simulink model "gm_NewSignalGenerator"  (R2026a)
settings: Solver=VariableStepAuto  StopTime=20e-4
libraries: dsphdlxfrm2 x1, simulink x1
settings Model: Creator=adams
settings OptimizationCC: ConditionallyExecuteInputs=off
settings DebuggingCC: InheritedTsInSrcMsg=none

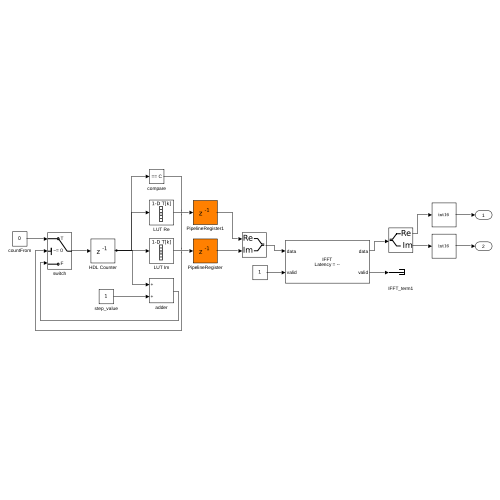
[thumbnail: Simulink's stored preview of the top-level diagram]
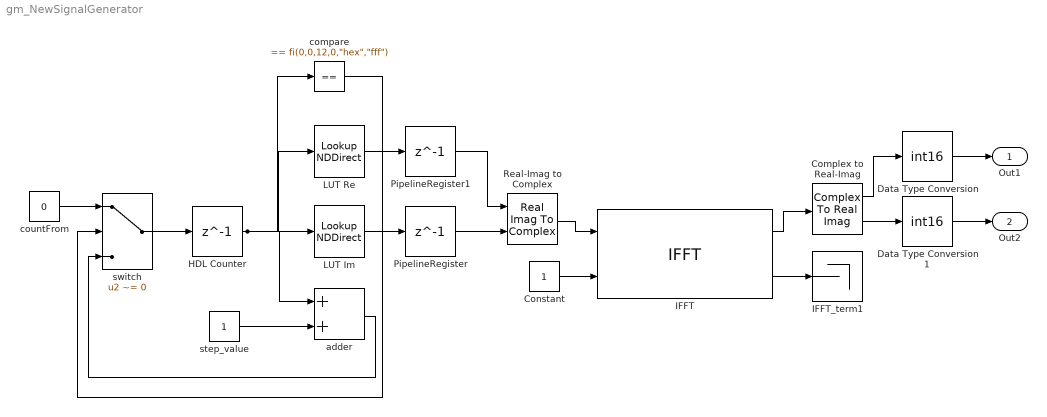
== system gm_NewSignalGenerator ==
  Complex to Real-Imag : ComplexToRealImag  SampleTime=6.51041666666667e-09
  Constant : Constant  OutDataTypeStr=boolean  SampleTime=6.51041666666667e-09
  Data Type Conversion : DataTypeConversion  OutDataTypeStr=int16  SampleTime=6.51041666666667e-09  SaturateOnIntegerOverflow=off  RndMeth=Floor
  Data Type Conversion1 : DataTypeConversion  OutDataTypeStr=int16  SampleTime=6.51041666666667e-09  SaturateOnIntegerOverflow=off  RndMeth=Floor
  HDL Counter : Delay  DelayLength=1  InitialCondition=0  SampleTime=6.51041666666667e-09
  IFFT : dsphdlxfrm2/IFFT  Architecture=Streaming Radix 2^2  FFTLengthSource=Property  FFTLength=4096  FFTLengthMax=1024  ComplexMultiplication=Use 4 multipliers and 2 adders  BitReversedOutput=off  BitReversedInput=off  Normalize=off  SimulateUsing=Code generation  RoundingMethod=Floor  ResetInputPort=off  StartOutputPort=off  EndOutputPort=off
  IFFT_term1 : Terminator
  LUT Im : LookupNDDirect  NumberOfTableDimensions=1  Table="reshape(double([0;0;0;0;0;0;0;0;-9;0;0;0;0;0;0;0;35;0;0;0;0;0;0;0;-78;0;0;0;0;0;0;0;138;0;0;0;0;0;0;0;-215;0;0;0;0;0;0;0;307;0;0;0;0;0;0;0;-413;0;0;0;0;0;0;0;530;0;0;0;0;0;0;0;-654;0;0;0;0;0;0;0;778;0;0;0;0;0;0;0;-895;0;0;0;0;0;0;0;995;0;0;0;0;0;0;0;-1068;0;0;0;0;0;0;0;1099;0;0;0;0;0;0;0;-1079;0;0;0;0;0;0;0;995;0;0;0;0;0;0;0;-842;0;0;0;0;0;0;0;618;0;0;0;0;0;0;0;-332;0;0;0;0;0;0;0;0;0;0;0;0;0;0;0;348;0;0;0;0;0;0;0;-674;0;0;0;0;0;0;0;933;0;0;0;0;0;0;0;-1081;0;0;0;0;0;0;0;1079;0;0;0;0;0;0;0;-910;0;0;0;0;0;0;0;582;0;0;0;0;0;0;0;-138;0;0;0;0;0;0;0;-348;0;0;0;0;0;0;0;778;0;0;0;0;0;0;0;-1049;0;0;0;0;0;0;0;1081;0;0;0;0;0;0;0;-842;0;0;0;0;0;0;0;373;0;0;0;0;0;0;0;215;0;0;0;0;0;0;0;-753;0;0;0;0;0;0;0;1068;0;0;0;0;0;0;0;-1035;0;0;0;0;0;0;0;640;0;0;0;0;0;0;0;0;0;0;0;0;0;0;0;-654;0;0;0;0;0;0;0;1056;0;0;0;0;0;0;0;-1020;0;0;0;0;0;0;0;530;0;0;0;0;0;0;0;215;0;0;0;0;0;0;0;-869;0;0;0;0;0;0;0;1097;0;0;0;0;0;0;0;-753;0;0;0;0;0;0;0;-9;0;0;0;0;0;0;0;778;0;0;0;0;0;0;0;-1100;0;0;0;0;0;0;0;753;0;0;0;0;0;0;0;78;0;0;0;0;0;0;0;-869;0;0;0;0;0;0;0;1079;0;0;0;0;0;0;0;-530;0;0;0;0;0;0;0;-413;0;0;0;0;0;0;0;1056;0;0;0;0;0;0;0;-885;0;0;0;0;0;0;0;0;0;0;0;0;0;0;0;895;0;0;0;0;0;0;0;-1035;0;0;0;0;0;0;0;265;0;0;0;0;0;0;0;753;0;0;0;0;0;0;0;-1079;0;0;0;0;0;0;0;373;0;0;0;0;0;0;0;708;0;0;0;0;0;0;0;-1081;0;0;0;0;0;0;0;332;0;0;0;0;0;0;0;778;0;0;0;0;0;0;0;-1043;0;0;0;0;0;0;0;138;0;0;0;0;0;0;0;933;0;0;0;0;0;0;0;-910;0;0;0;0;0;0;0;-215;0;0;0;0;0;0;0;1081;0;0;0;0;0;0;0;-582;0;0;0;0;0;0;0;-674;0;0;0;0;0;0;0;1043;0;0;0;0;0;0;0;0;0;0;0;0;0;0;0;-1049;0;0;0;0;0;0;0;618;0;0;0;0;0;0;0;708;0;0;0;0;0;0;0;-995;0;0;0;0;0;0;0;-215;0;0;0;0;0;0;0;1099;0;0;0;0;0;0;0;-265;0;0;0;0;0;0;0;-995;0;0;0;0;0;0;0;640;0;0;0;0;0;0;0;778;0;0;0;0;0;0;0;-885;0;0;0;0;0;0;0;-530;0;0;0;0;0;0;0;1020;0;0;0;0;0;0;0;307;0;0;0;0;0;0;0;-1079;0;0;0;0;0;0;0;-138;0;0;0;0;0;0;0;1097;0;0;0;0;0;0;0;35;0;0;0;0;0;0;0;-1100;0;0;0;0;0;0;0;0;0;0;0;0;0;0;0;1100;0;0;0;0;0;0;0;35;0;0;0;0;0;0;0;-1097;0;0;0;0;0;0;0;-138;0;0;0;0;0;0;0;1079;0;0;0;0;0;0;0;307;0;0;0;0;0;0;0;-1020;0;0;0;0;0;0;0;-530;0;0;0;0;0;0;0;885;0;0;0;0;0;0;0;778;0;0;0;0;0;0;0;-640;0;0;0;0;0;0;0;-995;0;0;0;0;0;0;0;265;0;0;0;0;0;0;0;1099;0;0;0;0;0;0;0;215;0;0;0;0;0;0;0;-995;0;0;0;0;0;0;0;-708;0;0;0;0;0;0;0;618;0;0;0;0;0;0;0;1049;0;0;0;0;0;0;0;0;0;0;0;0;0;0;0;-1043;0;0;0;0;0;0;0;-674;0;0;0;0;0;0;0;582;0;0;0;0;0;0;0;1081;0;0;0;0;0;0;0;215;0;0;0;0;0;0;0;-910;0;0;0;0;0;0;0;-933;0;0;0;0;0;0;0;138;0;0;0;0;0;0;0;1043;0;0;0;0;0;0;0;778;0;0;0;0;0;0;0;-332;0;0;0;0;0;0;0;-1081;0;0;0;0;0;0;0;-708;0;0;0;0;0;0;0;373;0;0;0;0;0;0;0;1079;0;0;0;0;0;0;0;753;0;0;0;0;0;0;0;-265;0;0;0;0;0;0;0;-1035;0;0;0;0;0;0;0;-895;0;0;0;0;0;0;0;0;0;0;0;0;0;0;0;885;0;0;0;0;0;0;0;1056;0;0;0;0;0;0;0;413;0;0;0;0;0;0;0;-530;0;0;0;0;0;0;0;-1079;0;0;0;0;0;0;0;-869;0;0;0;0;0;0;0;-78;0;0;0;0;0;0;0;753;0;0;0;0;0;0;0;1100;0;0;0;0;0;0;0;778;0;0;0;0;0;0;0;9;0;0;0;0;0;0;0;-753;0;0;0;0;0;0;0;-1097;0;0;0;0;0;0;0;-869;0;0;0;0;0;0;0;-215;0;0;0;0;0;0;0;530;0;0;0;0;0;0;0;1020;0;0;0;0;0;0;0;1056;0;0;0;0;0;0;0;654;0;0;0;0;0;0;0;0;0;0;0;0;0;0;0;-640;0;0;0;0;0;0;0;-1035;0;0;0;0;0;0;0;-1068;0;0;0;0;0;0;0;-753;0;0;0;0;0;0;0;-215;0;0;0;0;0;0;0;373;0;0;0;0;0;0;0;842;0;0;0;0;0;0;0;1081;0;0;0;0;0;0;0;1049;0;0;0;0;0;0;0;778;0;0;0;0;0;0;0;348;0;0;0;0;0;0;0;-138;0;0;0;0;0;0;0;-582;0;0;0;0;0;0;0;-910;0;0;0;0;0;0;0;-1079;0;0;0;0;0;0;0;-1081;0;0;0;0;0;0;0;-933;0;0;0;0;0;0;0;-674;0;0;0;0;0;0;0;-348;0;0;0;0;0;0;0;0;0;0;0;0;0;0;0;332;0;0;0;0;0;0;0;618;0;0;0;0;0;0;0;842;0;0;0;0;0;0;0;995;0;0;0;0;0;0;0;1079;0;0;0;0;0;0;0;1099;0;0;0;0;0;0;0;1068;0;0;0;0;0;0;0;995;0;0;0;0;0;0;0;895;0;0;0;0;0;0;0;778;0;0;0;0;0;0;0;654;0;0;0;0;0;0;0;530;0;0;0;0;0;0;0;413;0;0;0;0;0;0;0;307;0;0;0;0;0;0;0;215;0;0;0;0;0;0;0;138;0;0;0;0;0;0;0;78;0;0;0;0;0;0;0;35;0;0;0;0;0;0;0;9;0;0;0;0;0;0;0;0;0;0;0;0;0;0;0;0;0;0;0;0;0;0;0;0;0;0;0;0;0;0;0;0;0;0;0;0;0;0;0;0;0;0;0;0;0;0;0;0;0;0;0;0;0;0;0;0;0;0;0;0;0;0;0;0;0;0;0;0;0;0;0;0;0;0;0;0;0;0;0;0;0;0;0;0;0;0;0;0;0;0;0;0;0;0;0;0;0;0;0;0;0;0;0;0;0;0;0;0;0;0;0;0;0;0;0;0;0;0;0;0;0;0;0;0;0;0;0;0;0;0;0;0;0;0;0;0;0;0;0;0;0;0;0;0;0;0;0;0;0;0;0;0;0;0 ...(+5202 chars)]), [4096     1])"  SampleTime=6.51041666666667e-09  TableDataTypeStr=fixdt(1,32,20)
  LUT Re : LookupNDDirect  NumberOfTableDimensions=1  Table="reshape(double([1100;0;0;0;0;0;0;0;-1100;0;0;0;0;0;0;0;1099;0;0;0;0;0;0;0;-1097;0;0;0;0;0;0;0;1091;0;0;0;0;0;0;0;-1079;0;0;0;0;0;0;0;1056;0;0;0;0;0;0;0;-1020;0;0;0;0;0;0;0;964;0;0;0;0;0;0;0;-885;0;0;0;0;0;0;0;778;0;0;0;0;0;0;0;-640;0;0;0;0;0;0;0;468;0;0;0;0;0;0;0;-265;0;0;0;0;0;0;0;35;0;0;0;0;0;0;0;215;0;0;0;0;0;0;0;-468;0;0;0;0;0;0;0;708;0;0;0;0;0;0;0;-910;0;0;0;0;0;0;0;1049;0;0;0;0;0;0;0;-1100;0;0;0;0;0;0;0;1043;0;0;0;0;0;0;0;-869;0;0;0;0;0;0;0;582;0;0;0;0;0;0;0;-206;0;0;0;0;0;0;0;-215;0;0;0;0;0;0;0;618;0;0;0;0;0;0;0;-933;0;0;0;0;0;0;0;1091;0;0;0;0;0;0;0;-1043;0;0;0;0;0;0;0;778;0;0;0;0;0;0;0;-332;0;0;0;0;0;0;0;-206;0;0;0;0;0;0;0;708;0;0;0;0;0;0;0;-1035;0;0;0;0;0;0;0;1079;0;0;0;0;0;0;0;-802;0;0;0;0;0;0;0;265;0;0;0;0;0;0;0;373;0;0;0;0;0;0;0;-895;0;0;0;0;0;0;0;1100;0;0;0;0;0;0;0;-885;0;0;0;0;0;0;0;307;0;0;0;0;0;0;0;413;0;0;0;0;0;0;0;-964;0;0;0;0;0;0;0;1079;0;0;0;0;0;0;0;-674;0;0;0;0;0;0;0;-78;0;0;0;0;0;0;0;802;0;0;0;0;0;0;0;-1100;0;0;0;0;0;0;0;778;0;0;0;0;0;0;0;9;0;0;0;0;0;0;0;-802;0;0;0;0;0;0;0;1097;0;0;0;0;0;0;0;-674;0;0;0;0;0;0;0;-215;0;0;0;0;0;0;0;964;0;0;0;0;0;0;0;-1020;0;0;0;0;0;0;0;307;0;0;0;0;0;0;0;654;0;0;0;0;0;0;0;-1100;0;0;0;0;0;0;0;640;0;0;0;0;0;0;0;373;0;0;0;0;0;0;0;-1068;0;0;0;0;0;0;0;802;0;0;0;0;0;0;0;215;0;0;0;0;0;0;0;-1035;0;0;0;0;0;0;0;842;0;0;0;0;0;0;0;206;0;0;0;0;0;0;0;-1049;0;0;0;0;0;0;0;778;0;0;0;0;0;0;0;348;0;0;0;0;0;0;0;-1091;0;0;0;0;0;0;0;582;0;0;0;0;0;0;0;618;0;0;0;0;0;0;0;-1079;0;0;0;0;0;0;0;206;0;0;0;0;0;0;0;933;0;0;0;0;0;0;0;-869;0;0;0;0;0;0;0;-348;0;0;0;0;0;0;0;1100;0;0;0;0;0;0;0;-332;0;0;0;0;0;0;0;-910;0;0;0;0;0;0;0;842;0;0;0;0;0;0;0;468;0;0;0;0;0;0;0;-1079;0;0;0;0;0;0;0;35;0;0;0;0;0;0;0;1068;0;0;0;0;0;0;0;-468;0;0;0;0;0;0;0;-895;0;0;0;0;0;0;0;778;0;0;0;0;0;0;0;654;0;0;0;0;0;0;0;-964;0;0;0;0;0;0;0;-413;0;0;0;0;0;0;0;1056;0;0;0;0;0;0;0;215;0;0;0;0;0;0;0;-1091;0;0;0;0;0;0;0;-78;0;0;0;0;0;0;0;1099;0;0;0;0;0;0;0;9;0;0;0;0;0;0;0;-1100;0;0;0;0;0;0;0;-9;0;0;0;0;0;0;0;1099;0;0;0;0;0;0;0;78;0;0;0;0;0;0;0;-1091;0;0;0;0;0;0;0;-215;0;0;0;0;0;0;0;1056;0;0;0;0;0;0;0;413;0;0;0;0;0;0;0;-964;0;0;0;0;0;0;0;-654;0;0;0;0;0;0;0;778;0;0;0;0;0;0;0;895;0;0;0;0;0;0;0;-468;0;0;0;0;0;0;0;-1068;0;0;0;0;0;0;0;35;0;0;0;0;0;0;0;1079;0;0;0;0;0;0;0;468;0;0;0;0;0;0;0;-842;0;0;0;0;0;0;0;-910;0;0;0;0;0;0;0;332;0;0;0;0;0;0;0;1100;0;0;0;0;0;0;0;348;0;0;0;0;0;0;0;-869;0;0;0;0;0;0;0;-933;0;0;0;0;0;0;0;206;0;0;0;0;0;0;0;1079;0;0;0;0;0;0;0;618;0;0;0;0;0;0;0;-582;0;0;0;0;0;0;0;-1091;0;0;0;0;0;0;0;-348;0;0;0;0;0;0;0;778;0;0;0;0;0;0;0;1049;0;0;0;0;0;0;0;206;0;0;0;0;0;0;0;-842;0;0;0;0;0;0;0;-1035;0;0;0;0;0;0;0;-215;0;0;0;0;0;0;0;802;0;0;0;0;0;0;0;1068;0;0;0;0;0;0;0;373;0;0;0;0;0;0;0;-640;0;0;0;0;0;0;0;-1100;0;0;0;0;0;0;0;-654;0;0;0;0;0;0;0;307;0;0;0;0;0;0;0;1020;0;0;0;0;0;0;0;964;0;0;0;0;0;0;0;215;0;0;0;0;0;0;0;-674;0;0;0;0;0;0;0;-1097;0;0;0;0;0;0;0;-802;0;0;0;0;0;0;0;-9;0;0;0;0;0;0;0;778;0;0;0;0;0;0;0;1100;0;0;0;0;0;0;0;802;0;0;0;0;0;0;0;78;0;0;0;0;0;0;0;-674;0;0;0;0;0;0;0;-1079;0;0;0;0;0;0;0;-964;0;0;0;0;0;0;0;-413;0;0;0;0;0;0;0;307;0;0;0;0;0;0;0;885;0;0;0;0;0;0;0;1100;0;0;0;0;0;0;0;895;0;0;0;0;0;0;0;373;0;0;0;0;0;0;0;-265;0;0;0;0;0;0;0;-802;0;0;0;0;0;0;0;-1079;0;0;0;0;0;0;0;-1035;0;0;0;0;0;0;0;-708;0;0;0;0;0;0;0;-206;0;0;0;0;0;0;0;332;0;0;0;0;0;0;0;778;0;0;0;0;0;0;0;1043;0;0;0;0;0;0;0;1091;0;0;0;0;0;0;0;933;0;0;0;0;0;0;0;618;0;0;0;0;0;0;0;215;0;0;0;0;0;0;0;-206;0;0;0;0;0;0;0;-582;0;0;0;0;0;0;0;-869;0;0;0;0;0;0;0;-1043;0;0;0;0;0;0;0;-1100;0;0;0;0;0;0;0;-1049;0;0;0;0;0;0;0;-910;0;0;0;0;0;0;0;-708;0;0;0;0;0;0;0;-468;0;0;0;0;0;0;0;-215;0;0;0;0;0;0;0;35;0;0;0;0;0;0;0;265;0;0;0;0;0;0;0;468;0;0;0;0;0;0;0;640;0;0;0;0;0;0;0;778;0;0;0;0;0;0;0;885;0;0;0;0;0;0;0;964;0;0;0;0;0;0;0;1020;0;0;0;0;0;0;0;1056;0;0;0;0;0;0;0;1079;0;0;0;0;0;0;0;1091;0;0;0;0;0;0;0;1097;0;0;0;0;0;0;0;1099;0;0;0;0;0;0;0;1100;0;0;0;0;0;0;0;0;0;0;0;0;0;0;0;0;0;0;0;0;0;0;0;0;0;0;0;0;0;0;0;0;0;0;0;0;0;0;0;0;0;0;0;0;0;0;0;0;0;0;0;0;0;0;0;0;0;0;0;0;0;0;0;0;0;0;0;0;0;0;0;0;0;0;0;0;0;0;0;0;0;0;0;0;0;0;0;0;0;0;0;0;0;0;0;0;0;0;0;0;0;0;0;0;0;0;0;0;0;0;0;0;0;0;0;0;0;0;0;0;0;0;0;0;0;0;0;0;0;0;0;0;0;0;0;0;0 ...(+5271 chars)]), [4096     1])"  SampleTime=6.51041666666667e-09  TableDataTypeStr=fixdt(1,32,20)
  PipelineRegister : Delay  DelayLength=1  InitialCondition=0  SampleTime=6.51041666666667e-09
  PipelineRegister1 : Delay  DelayLength=1  InitialCondition=0  SampleTime=6.51041666666667e-09
  Real-Imag to Complex : RealImagToComplex  ConstantPart="fi(0,1,32,20,\"hex\",\"00000000\")"  SampleTime=6.51041666666667e-09
  adder : Sum  OutDataTypeStr=fixdt(0, 12, 0)  AccumDataTypeStr=fixdt(0, 12, 0)  SampleTime=6.51041666666667e-09
  compare : simulink/Logic and Bit Operations/Compare To Constant  relop===  const="fi(0,0,12,0,\"hex\",\"fff\")"  OutDataTypeStr=boolean
  countFrom : Constant  Value=0  VectorParams1D=off  OutDataTypeStr=fixdt(0, 12, 0)  SampleTime=6.51041666666667e-09
  step_value : Constant  VectorParams1D=off  OutDataTypeStr=fixdt(0, 12, 0)  SampleTime=6.51041666666667e-09
  switch : Switch  Criteria=u2 ~= 0  Threshold="fi(0,0,1,0,\"hex\",\"0\")"  OutDataTypeStr=fixdt(0, 12, 0)  SampleTime=6.51041666666667e-09  SaturateOnIntegerOverflow=off  InputSameDT=off
  Out1 : Outport  SampleTime=6.51041666666667e-09
  Out2 : Outport  Port=2  SampleTime=6.51041666666667e-09
  wires:
  Data Type Conversion1/1 -> Out2/1
  Complex to Real-Imag/2 -> Data Type Conversion1/1
  Data Type Conversion/1 -> Out1/1
  IFFT/2 -> IFFT_term1/1
  countFrom/1 -> switch/1
  switch/1 -> HDL Counter/1
  step_value/1 -> adder/2
  LUT Im/1 -> PipelineRegister/1
  HDL Counter/1 -> compare/1, adder/1, LUT Im/1, LUT Re/1
  PipelineRegister/1 -> Real-Imag to Complex/2
  compare/1 -> switch/2
  PipelineRegister1/1 -> Real-Imag to Complex/1
  IFFT/1 -> Complex to Real-Imag/1
  LUT Re/1 -> PipelineRegister1/1
  Complex to Real-Imag/1 -> Data Type Conversion/1
  Real-Imag to Complex/1 -> IFFT/1
  adder/1 -> switch/3
  Constant/1 -> IFFT/2
